simulink model "Lab6_ciagly"  (R2017a)
settings: Solver=FixedStepAuto  StartTime=0.0  StopTime=10.0  FixedStep=0.01  RelTol=1e-3
libraries: cstblocks x2
settings Model: Creator=ishiguro  LastModifiedBy=ishiguro

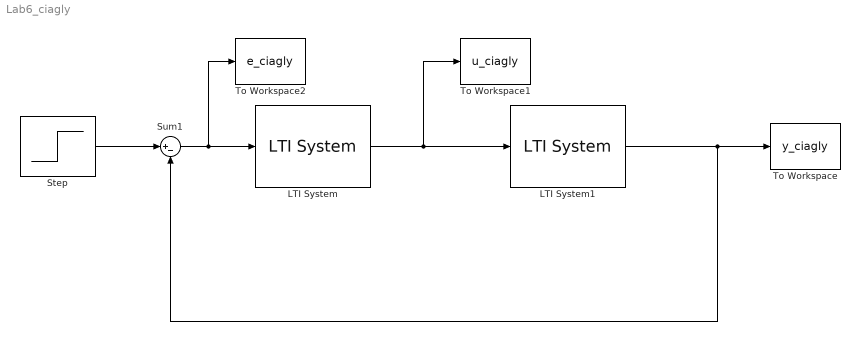
== system Lab6_ciagly ==
  LTI System : cstblocks/LTI System  sys=Kr  IC=[]
  LTI System1 : cstblocks/LTI System  sys=K  IC=[]
  Step : Step  Time=0  SampleTime=0
  Sum1 : Sum  Inputs=|+-
  To Workspace : ToWorkspace  VariableName=y_ciagly  SampleTime=-1
  To Workspace1 : ToWorkspace  VariableName=u_ciagly  SampleTime=-1
  To Workspace2 : ToWorkspace  VariableName=e_ciagly  SampleTime=-1
  wires:
  Step/1 -> Sum1/1
  LTI System1/1 -> To Workspace/1, Sum1/2
  LTI System/1 -> To Workspace1/1, LTI System1/1
  Sum1/1 -> To Workspace2/1, LTI System/1
